simulink model "sim_mpc_ex2"  (R2025b)
settings: Solver=ode45  StartTime=0.0  StopTime=t_sim  MaxStep=1e-3*Ts  MinStep=1e-4*Ts  RelTol=1e-3
undefined symbols (not defined in the file): C, md, Ts
libraries: cstblocks x1
settings Model: Creator=davidecovolo  LastModifiedBy=davidecovolo
settings SolverCC: InitialStep=1e-4*Ts

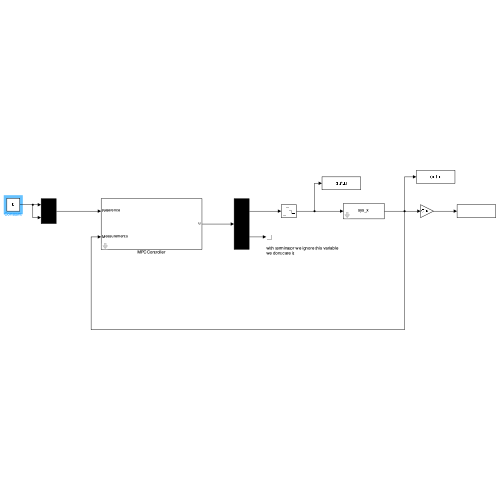
[thumbnail: Simulink's stored preview of the top-level diagram]
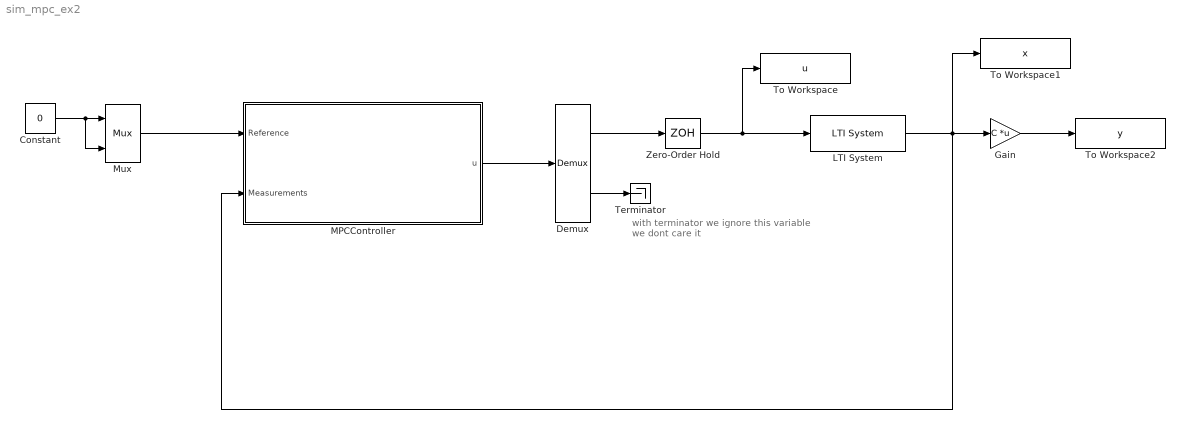
== system sim_mpc_ex2 ==
  note: with terminator we ignore this variable
      | we dont care it
  Constant : Constant  Value=0
  Demux : Demux  Outputs=2
  Gain : Gain  Gain=C  Multiplication=Matrix(K*u)
  LTI System : cstblocks/LTI System  sys=sys_x  IC=x0  PadeOrder=0
  MPCController : Subsystem  mask{md=md}
      mask prompts: md "MPCData"
  Mux : Mux  Inputs=2
  Terminator : Terminator
  To Workspace : ToWorkspace  VariableName=u  SaveFormat=Timeseries  SampleTime=Ts
  To Workspace1 : ToWorkspace  VariableName=x  SaveFormat=Timeseries  SampleTime=Ts
  To Workspace2 : ToWorkspace  VariableName=y  SaveFormat=Timeseries  SampleTime=Ts
  Zero-Order Hold : ZeroOrderHold  SampleTime=Ts
  wires:
  Mux/1 -> MPCController/1(Reference)
  Gain/1 -> To Workspace2/1
  LTI System/1 -> To Workspace1/1, MPCController/2(Measurements), Gain/1
  Zero-Order Hold/1 -> LTI System/1, To Workspace/1
  MPCController/1(u) -> Demux/1
  Demux/1 -> Zero-Order Hold/1
  Demux/2 -> Terminator/1
  Constant/1 -> Mux/2, Mux/1

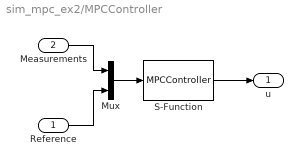
== system sim_mpc_ex2/MPCController ==
  Reference : Inport
  Measurements : Inport  Port=2
  Mux : Mux  Inputs=2
  S-Function : S-Function  FunctionName=MPCController  Parameters=md  SFunctionDeploymentMode=off  EnableBusSupport=off
  u : Outport
  wires:
  Mux/1 -> S-Function/1
  Measurements/1 -> Mux/1
  Reference/1 -> Mux/2
  S-Function/1 -> u/1
